simulink model "Washingmachine"  (R2022b)
settings: Solver=VariableStepAuto  StartTime=0.0  StopTime=45  RelTol=1e-3
settings Model: Creator=AKHIL  LastModifiedBy=AKHIL

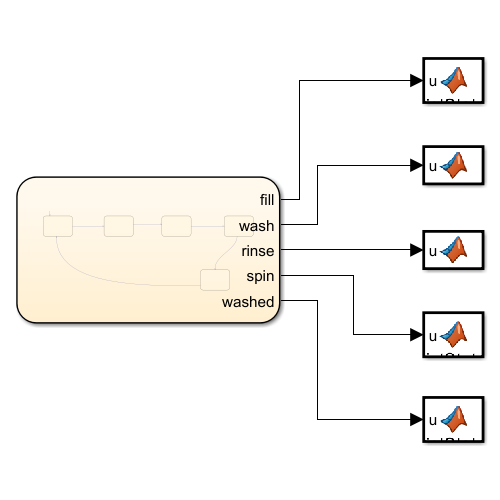
[thumbnail: Simulink's stored preview of the top-level diagram]
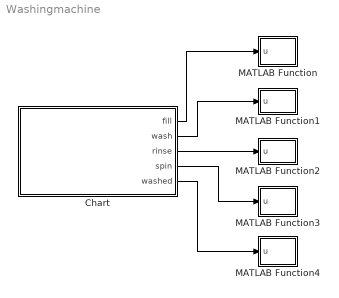
== system Washingmachine ==
  Chart : Stateflow chart  TreatAsAtomicUnit=on
  MATLAB Function : MATLAB Function  TreatAsAtomicUnit=on
  MATLAB Function1 : MATLAB Function  TreatAsAtomicUnit=on
  MATLAB Function2 : MATLAB Function  TreatAsAtomicUnit=on
  MATLAB Function3 : MATLAB Function  TreatAsAtomicUnit=on
  MATLAB Function4 : MATLAB Function  TreatAsAtomicUnit=on
  wires:
  Chart/2(wash) -> MATLAB Function1/1(u)
  Chart/3(rinse) -> MATLAB Function2/1(u)
  Chart/4(spin) -> MATLAB Function3/1(u)
  Chart/5(washed) -> MATLAB Function4/1(u)
  Chart/1(fill) -> MATLAB Function/1(u)

== matlab function Washingmachine/MATLAB Function1 ==
  data: u input
function printStatus(u)
    if u == 1
        disp("Washing");
    else
        disp("");
    end
end

== matlab function Washingmachine/MATLAB Function ==
  data: u input
function printStatus(u)
    if u == 1
        disp("Fill the machine");
    else
        disp("");
    end
end

== stateflow chart Washingmachine/Chart ==
  state Fill
    entry:
    washed=0;
    during:
    fill=1;
  state Wash
    entry:
    fill=0;
    during:
    wash=1;
  state Rinse
    entry:
    wash=0;
    during:
    rinse=1;
  state Spin
    entry:
    rinse=0;
    during:
    spin=1;
  state Done
    entry:
    spin=0;
    during:
    washed=1;
  (default) -> Fill
  Wash -> Rinse : [after(20,sec)]
  Fill -> Wash : [after(10,sec)]
  Rinse -> Spin : [after(5,sec)]
  Done -> Fill : [after(1,sec)]
  Spin -> Done : [after(5,sec)]
  data: fill output; wash output; rinse output; spin output; washed output

== matlab function Washingmachine/MATLAB Function2 ==
  data: u input
function printStatus(u)
    if u == 1
        disp("Rinsing");
    else
        disp("");
    end
end

== matlab function Washingmachine/MATLAB Function3 ==
  data: u input
function printStatus(u)
    if u == 1
        disp("Spinning");
    else
        disp("");
    end
end

== matlab function Washingmachine/MATLAB Function4 ==
  data: u input
function printStatus(u)
    if u == 1
        disp("Washed");
    else
        disp("");
    end
end
